simulink model "cap_array"  (R2014a)
settings: Solver=ode45  StartTime=0.0  StopTime=0.015  MaxStep=1e-5  RelTol=1e-3
values from neighbouring files (symbols this model uses):
  C = 4.6e-5    (= 4.6e-05)    [tipe_vars.m]
  K = (pi*Rproj^4*gam*(mu*n)^2)/(8*m*Rbob^2)    (= 2.96114824556e-08)    [tipe_vars.m]
  L0 = 0.0015    [tipe_vars.m]
  Lbob = 0.06    [tipe_vars.m]
  Lproj = 0.025    [tipe_vars.m]
  R = 15    [tipe_vars.m]
  Rbob = 0.015    [tipe_vars.m]
  U0 = 800    [tipe_vars.m]
settings Model: Creator=jackhalford  LastModifiedBy=jackhalford
settings SolverCC: ShapePreserveControl=EnableAll  ZeroCrossControl=DisableAll

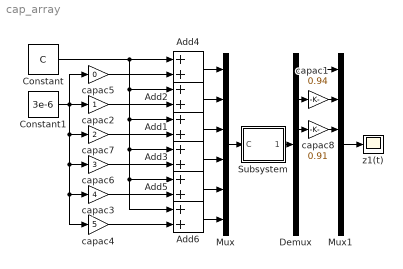
== system cap_array ==
  Add{1..6} (6 alike) : Sum
  Constant : Constant  Value=C
  Constant1 : Constant  Value=3e-6
  Demux : Demux  Outputs=6
  Mux : Mux  Inputs=6
  Mux1 : Mux  Inputs=6
  Subsystem : Subsystem
  capac1 : Gain  Gain=0.94
  capac2 : Gain
  capac3 : Gain  Gain=4
  capac4 : Gain  Gain=5
  capac5 : Gain  Gain=0
  capac6 : Gain  Gain=3
  capac7 : Gain  Gain=2
  capac8 : Gain  Gain=0.91
  "z1(t) " : Scope
      settings: TickLabels=on  TimeRange=0.007  YMin=0  YMax=45  SaveName=ScopeData14
  wires:
  Add4/1 -> Mux/1
  Add2/1 -> Mux/2
  Constant/1 -> Add1/1, Add6/1, Add5/1, Add3/1, Add2/1, Add4/1
  Constant1/1 -> capac7/1, capac6/1, capac4/1, capac3/1, capac2/1, capac5/1
  capac5/1 -> Add4/2
  capac2/1 -> Add2/2
  capac7/1 -> Add1/2
  capac6/1 -> Add3/2
  capac3/1 -> Add5/2
  capac4/1 -> Add6/2
  Mux/1 -> Subsystem/1(C)
  Add1/1 -> Mux/3
  Add3/1 -> Mux/4
  Add5/1 -> Mux/5
  Add6/1 -> Mux/6
  Subsystem/1(Out1) -> Demux/1
  Mux1/1 -> "z1(t) "/1
  Demux/1 -> Mux1/1
  capac1/1 -> Mux1/2
  Demux/2 -> capac1/1
  Demux/3 -> capac8/1
  capac8/1 -> Mux1/3

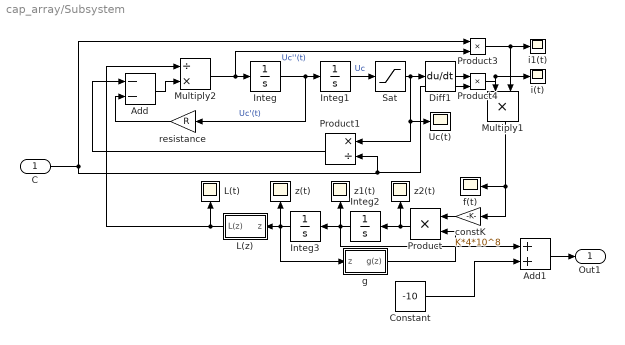
== system cap_array/Subsystem ==
  C : Inport
  Add : Sum  Inputs=--
  Add1 : Sum
  Constant : Constant  Value=-10
  Diff1 : Derivative
  Integ : Integrator
  "Integ1 " : Integrator  InitialCondition=-U0
  Integ2 : Integrator  InitialCondition=10
  Integ3 : Integrator  InitialCondition=-(Lbob+Lproj)/2
  L(t) : Scope
      settings: TimeRange=0.003  YMin=-0.0425  YMax=-0.04235
  L(z) : Subsystem
  Multiply1 : Product  Inputs=**
  Multiply2 : Product  Inputs=/*
  Product : Product  Inputs=**
  Product1 : Product  Inputs=*/
  Product3 : Product  Inputs=**
  Product4 : Product  Inputs=**
  Sat : Saturate  UpperLimit=10000  LowerLimit=-10000
  Uc(t) : Scope
      settings: ShowLegends=on  TimeRange=0.001  YMin=-800  YMax=-799.963
  constK : Gain  Gain=K*4*10^8
  f(t) : Scope
      settings: TimeRange=0.005  YMin=0  YMax=80  SaveName=ScopeData6
  g : Subsystem
  i(t) : Scope
      settings: TimeRange=0.005  YMin=0  YMax=80  SaveName=ScopeData17
  i1(t) : Scope
      settings: YMin=-180  YMax=-155  SaveName=ScopeData16
  resistance : Gain  Gain=R
  z(t) : Scope
      settings: TimeRange=0.003  YMin=-0.0425  YMax=-0.04235  SaveName=ScopeData4
  z1(t) : Scope
      settings: TimeRange=0.03  YMin=0  YMax=120  SaveName=ScopeData13
  z2(t) : Scope
      settings: YMin=1.03225e-09  YMax=1.03675e-09  SaveName=ScopeData3
  Out1 : Outport
  wires:
  Product4/1 -> i(t)/1, Multiply1/1
  Multiply2/1 -> Product3/2, Integ/1  "Uc''(t)"
  Integ/1 -> resistance/1, "Integ1 "/1  "Uc'(t)"
  resistance/1 -> Add/2
  Add/1 -> Multiply2/2
  Product1/1 -> Add/1
  Diff1/1 -> Product4/1
  "Integ1 "/1 -> Sat/1  "Uc"
  Sat/1 -> Diff1/1, Product1/1, Uc(t)/1
  Product/1 -> Integ2/1, z2(t)/1
  Integ2/1 -> z1(t)/1, Add1/1, Integ3/1
  Integ3/1 -> g/1("z "), L(z)/1("z "), z(t)/1
  Product3/1 -> i1(t)/1, Multiply1/2
  Multiply1/1 -> constK/1, f(t)/1
  constK/1 -> Product/1
  g/1(g(z)) -> Product/2
  L(z)/1(L(z)) -> Multiply2/1, L(t)/1
  C/1 -> Product4/2, Product1/2, Product3/1
  Add1/1 -> Out1/1
  Constant/1 -> Add1/2

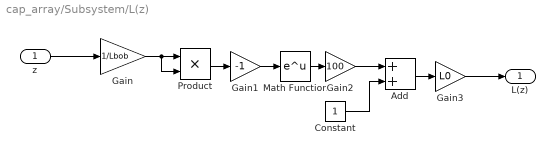
== system cap_array/Subsystem/L(z) ==
  "z " : Inport
  Add : Sum
  Constant : Constant
  Gain : Gain  Gain=1/Lbob
  Gain1 : Gain  Gain=-1
  Gain2 : Gain  Gain=100
  Gain3 : Gain  Gain=L0
  Math Function : Math  SaturateOnIntegerOverflow=on
  Product : Product
  L(z) : Outport
  wires:
  "z "/1 -> Gain/1
  Gain/1 -> Product/2, Product/1
  Product/1 -> Gain1/1
  Gain1/1 -> Math Function/1
  Math Function/1 -> Gain2/1
  Gain2/1 -> Add/1
  Constant/1 -> Add/2
  Add/1 -> Gain3/1
  Gain3/1 -> L(z)/1

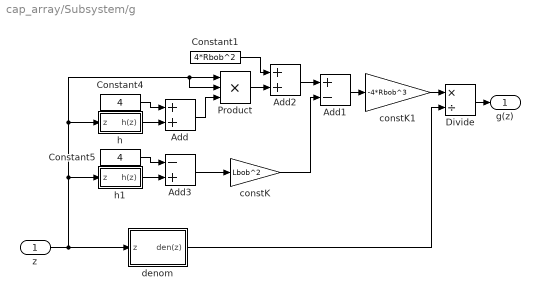
== system cap_array/Subsystem/g ==
  "z " : Inport
  Add : Sum
  Add1 : Sum  Inputs=+-
  Add2 : Sum
  Add3 : Sum  Inputs=-+
  Constant1 : Constant  Value=4*Rbob^2
  Constant4 : Constant  Value=4
  Constant5 : Constant  Value=4
  Divide : Product  Inputs=*/
  Product : Product  Inputs=3
  constK : Gain  Gain=Lbob^2
  constK1 : Gain  Gain=-4*Rbob^3
  denom : Subsystem
  "h " : Subsystem
  "h1 " : Subsystem
  g(z) : Outport
  wires:
  Add/1 -> Product/3
  "h "/1(h(z)) -> Add/2
  Add2/1 -> Add1/1
  Divide/1 -> g(z)/1
  "z "/1 -> denom/1("z "), "h "/1("z "), Product/2, Product/1, "h1 "/1("z ")
  Constant4/1 -> Add/1
  Product/1 -> Add2/2
  Constant1/1 -> Add2/1
  constK/1 -> Add1/2
  denom/1(den(z)) -> Divide/2
  Constant5/1 -> Add3/1
  "h1 "/1(h(z)) -> Add3/2
  Add3/1 -> constK/1
  constK1/1 -> Divide/1
  Add1/1 -> constK1/1

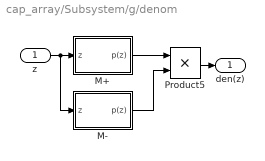
== system cap_array/Subsystem/g/denom ==
  "z " : Inport
  M+ : Subsystem
  M- : Subsystem
  Product5 : Product
  den(z) : Outport
  wires:
  "z "/1 -> M-/1("z "), M+/1("z ")
  M+/1(p(z)) -> Product5/1
  M-/1(p(z)) -> Product5/2
  Product5/1 -> den(z)/1

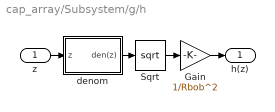
== system cap_array/Subsystem/g/h  ==
  "z " : Inport
  Gain : Gain  Gain=1/Rbob^2
  Sqrt : Sqrt  SaturateOnIntegerOverflow=on
  denom : Subsystem
  h(z) : Outport
  wires:
  "z "/1 -> denom/1("z ")
  denom/1(den(z)) -> Sqrt/1
  Sqrt/1 -> Gain/1
  Gain/1 -> h(z)/1

== system cap_array/Subsystem/g/h1  ==
  "z " : Inport
  Gain : Gain  Gain=1/Rbob^2
  Sqrt : Sqrt  SaturateOnIntegerOverflow=on
  denom : Subsystem
  h(z) : Outport
  wires:
  "z "/1 -> denom/1("z ")
  denom/1(den(z)) -> Sqrt/1
  Sqrt/1 -> Gain/1
  Gain/1 -> h(z)/1

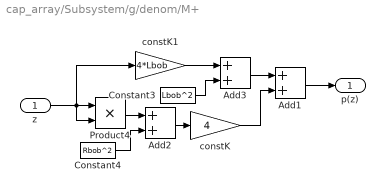
== system cap_array/Subsystem/g/denom/M+ ==
  "z " : Inport
  Add1 : Sum
  Add2 : Sum
  Add3 : Sum
  Constant3 : Constant  Value=Lbob^2
  Constant4 : Constant  Value=Rbob^2
  Product4 : Product
  constK : Gain  Gain=4
  constK1 : Gain  Gain=4*Lbob
  p(z) : Outport
  wires:
  Product4/1 -> Add2/1
  Constant4/1 -> Add2/2
  Add2/1 -> constK/1
  constK1/1 -> Add3/1
  Constant3/1 -> Add3/2
  "z "/1 -> constK1/1, Product4/2, Product4/1
  Add3/1 -> Add1/1
  constK/1 -> Add1/2
  Add1/1 -> p(z)/1

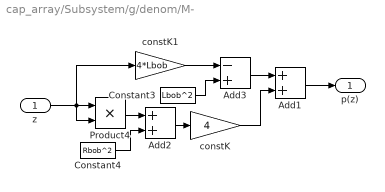
== system cap_array/Subsystem/g/denom/M- ==
  "z " : Inport
  Add1 : Sum
  Add2 : Sum
  Add3 : Sum  Inputs=-+
  Constant3 : Constant  Value=Lbob^2
  Constant4 : Constant  Value=Rbob^2
  Product4 : Product
  constK : Gain  Gain=4
  constK1 : Gain  Gain=4*Lbob
  p(z) : Outport
  wires:
  Product4/1 -> Add2/1
  Constant4/1 -> Add2/2
  Add2/1 -> constK/1
  constK1/1 -> Add3/1
  Constant3/1 -> Add3/2
  "z "/1 -> constK1/1, Product4/2, Product4/1
  Add3/1 -> Add1/1
  constK/1 -> Add1/2
  Add1/1 -> p(z)/1

== system cap_array/Subsystem/g/h /denom ==
  "z " : Inport
  M+ : Subsystem
  M- : Subsystem
  Product5 : Product
  den(z) : Outport
  wires:
  "z "/1 -> M-/1("z "), M+/1("z ")
  M+/1(p(z)) -> Product5/1
  M-/1(p(z)) -> Product5/2
  Product5/1 -> den(z)/1

== system cap_array/Subsystem/g/h1 /denom ==
  "z " : Inport
  M+ : Subsystem
  M- : Subsystem
  Product5 : Product
  den(z) : Outport
  wires:
  "z "/1 -> M-/1("z "), M+/1("z ")
  M+/1(p(z)) -> Product5/1
  M-/1(p(z)) -> Product5/2
  Product5/1 -> den(z)/1

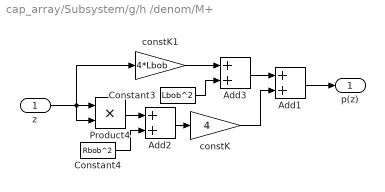
== system cap_array/Subsystem/g/h /denom/M+ ==
  "z " : Inport
  Add1 : Sum
  Add2 : Sum
  Add3 : Sum
  Constant3 : Constant  Value=Lbob^2
  Constant4 : Constant  Value=Rbob^2
  Product4 : Product
  constK : Gain  Gain=4
  constK1 : Gain  Gain=4*Lbob
  p(z) : Outport
  wires:
  Product4/1 -> Add2/1
  Constant4/1 -> Add2/2
  Add2/1 -> constK/1
  constK1/1 -> Add3/1
  Constant3/1 -> Add3/2
  "z "/1 -> constK1/1, Product4/2, Product4/1
  Add3/1 -> Add1/1
  constK/1 -> Add1/2
  Add1/1 -> p(z)/1

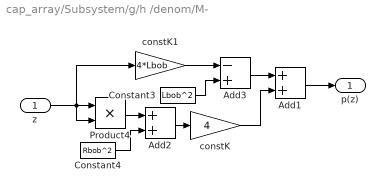
== system cap_array/Subsystem/g/h /denom/M- ==
  "z " : Inport
  Add1 : Sum
  Add2 : Sum
  Add3 : Sum  Inputs=-+
  Constant3 : Constant  Value=Lbob^2
  Constant4 : Constant  Value=Rbob^2
  Product4 : Product
  constK : Gain  Gain=4
  constK1 : Gain  Gain=4*Lbob
  p(z) : Outport
  wires:
  Product4/1 -> Add2/1
  Constant4/1 -> Add2/2
  Add2/1 -> constK/1
  constK1/1 -> Add3/1
  Constant3/1 -> Add3/2
  "z "/1 -> constK1/1, Product4/2, Product4/1
  Add3/1 -> Add1/1
  constK/1 -> Add1/2
  Add1/1 -> p(z)/1

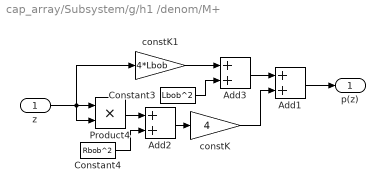
== system cap_array/Subsystem/g/h1 /denom/M+ ==
  "z " : Inport
  Add1 : Sum
  Add2 : Sum
  Add3 : Sum
  Constant3 : Constant  Value=Lbob^2
  Constant4 : Constant  Value=Rbob^2
  Product4 : Product
  constK : Gain  Gain=4
  constK1 : Gain  Gain=4*Lbob
  p(z) : Outport
  wires:
  Product4/1 -> Add2/1
  Constant4/1 -> Add2/2
  Add2/1 -> constK/1
  constK1/1 -> Add3/1
  Constant3/1 -> Add3/2
  "z "/1 -> constK1/1, Product4/2, Product4/1
  Add3/1 -> Add1/1
  constK/1 -> Add1/2
  Add1/1 -> p(z)/1

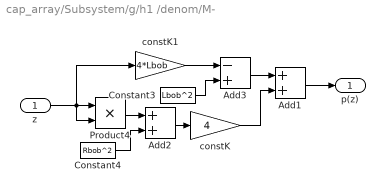
== system cap_array/Subsystem/g/h1 /denom/M- ==
  "z " : Inport
  Add1 : Sum
  Add2 : Sum
  Add3 : Sum  Inputs=-+
  Constant3 : Constant  Value=Lbob^2
  Constant4 : Constant  Value=Rbob^2
  Product4 : Product
  constK : Gain  Gain=4
  constK1 : Gain  Gain=4*Lbob
  p(z) : Outport
  wires:
  Product4/1 -> Add2/1
  Constant4/1 -> Add2/2
  Add2/1 -> constK/1
  constK1/1 -> Add3/1
  Constant3/1 -> Add3/2
  "z "/1 -> constK1/1, Product4/2, Product4/1
  Add3/1 -> Add1/1
  constK/1 -> Add1/2
  Add1/1 -> p(z)/1
